simulink model "tmp_model_3"  (R2018b)
settings: Solver=VariableStepAuto  StartTime=0.0  StopTime=100  FixedStep=0.001  RelTol=1e-3
undefined symbols (not defined in the file or in its folder): GeRa
libraries: fl_lib x63, sdl_lib x20, nesl_utility x11
(part 3 of 3)

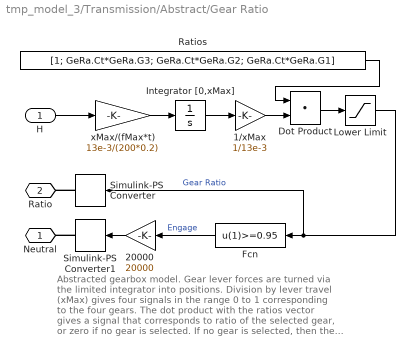
== system tmp_model_3/Transmission/Abstract/Gear Ratio ==
  note: Abstracted gearbox model. Gear lever forces are turned
      | via the limited integrator into positions. Division
      | by lever travel (xMax) gives four signals in the range
      | 0 to 1 corresponding to the four gears. The dot
      | product with the ratios vector gives a signal that
      | corresponds to ratio of the selected gear, or zero if
      | no gear is selected. If no gear is selected, then the
      | clutch is disengaged to represent neutral.
  H : Inport
  1/xMax : Gain  Gain=1/13e-3  SaturateOnIntegerOverflow=on  OutDataTypeStr=Inherit: Same as input  ParamDataTypeStr=Inherit: Same as input
  20000 : Gain  Gain=20000  SaturateOnIntegerOverflow=on  OutDataTypeStr=Inherit: Same as input  ParamDataTypeStr=Inherit: Same as input
  Dot Product : DotProduct  OutDataTypeStr=Inherit: Inherit via internal rule
  Fcn : Fcn  Expr=u(1)>=0.95
  Integrator [0,xMax] : Integrator  LimitOutput=on  UpperSaturationLimit=13e-3  LowerSaturationLimit=0
  Lower Limit : Saturate  UpperLimit=inf  LowerLimit=0.9
  Ratios : Constant  Value=[1; GeRa.Ct*GeRa.G3; GeRa.Ct*GeRa.G2; GeRa.Ct*GeRa.G1]  VectorParams1D=off
  Simulink-PS Converter : nesl_utility/Simulink-PS Converter  PhysicalDomain=network_engine_domain  SubClassName=ps_input  LeftPortType=input  RightPortType=output  PseudoPeriodic=off  Frequencies=[]  NoiseDistribution=none  NoiseParameters=[]  Unit=1  AffineConversion=off  FilteringAndDerivatives=zero  SimscapeFilterOrder=1  InputFilterTimeConstant=.001  UdotUserProvided=0
  Simulink-PS Converter1 : nesl_utility/Simulink-PS Converter  PhysicalDomain=network_engine_domain  SubClassName=ps_input  LeftPortType=input  RightPortType=output  PseudoPeriodic=off  Frequencies=[]  NoiseDistribution=none  NoiseParameters=[]  Unit=1  AffineConversion=off  FilteringAndDerivatives=zero  SimscapeFilterOrder=1  InputFilterTimeConstant=.001  UdotUserProvided=0
  xMax/(fMax*t) : Gain  Gain=13e-3/(200*0.2)  SaturateOnIntegerOverflow=on  OutDataTypeStr=Inherit: Same as input  ParamDataTypeStr=Inherit: Same as input
  Neutral : PMIOPort  Side=Right
  Ratio : PMIOPort  Port=2  Side=Right
  wires:
  Lower Limit/1 -> Fcn/1, Simulink-PS Converter/1  "Gear Ratio"
  20000/1 -> Simulink-PS Converter1/1
  Fcn/1 -> 20000/1  "Engage"
  xMax/(fMax*t)/1 -> Integrator [0,xMax]/1
  1/xMax/1 -> Dot Product/2
  Integrator [0,xMax]/1 -> 1/xMax/1
  Dot Product/1 -> Lower Limit/1
  H/1 -> xMax/(fMax*t)/1
  Ratios/1 -> Dot Product/1
  connections:
  Simulink-PS Converter1/RConn1 -- Neutral/RConn1
  Simulink-PS Converter/RConn1 -- Ratio/RConn1

== system tmp_model_3/Transmission/Detailed/Gearbox Schematic ==

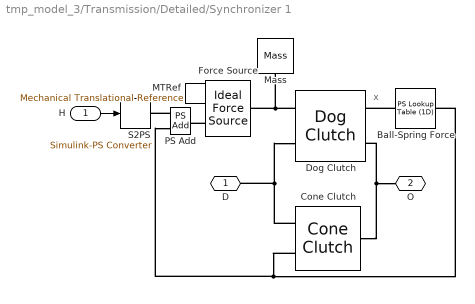
== system tmp_model_3/Transmission/Detailed/Synchronizer 1 ==
  note: x
  H : Inport
  Ball-Spring Force : fl_lib/Physical Signals/Lookup Tables/PS Lookup Table (1D)  x=[ -2 -0.1 0 0.1 2 ]*1e-3+3.2e-3  f=[ 0 100 0 -100 0 ]  interp_method=1  extrap_method=2
      settings: SourceProductName=Simscape  SourceProductBaseCode=SS
  Cone Clutch : sdl_lib/Clutches/Cone Clutch  d_o=60 mm  d_i=50 mm  theta=15 deg  friction_model=1  mu_coulomb=0.5  mu_w_vector=[ 0 0.1 0.2 0.3 0.4 0.5 1 2 5 10 100 1000 ] rad/s  mu_coulomb_vector=[ 0.29 0.28 0.26 0.22 0.21 0.2 0.2 0.19 0.19 0.19 0.19 0.19 ]  mu_interp_method=1  mu_extrap_method=1  mu_static=0.52  w_tol=0.01 rad/s  force_min=1 N  initial_state_locked=0  temperature_TLU=[280.0, 300.0, 320.0] K  mu_coulomb_temp_vector=[0.3, 0.28, 0.25]  mu_coulomb_matrix=[0.34, 0.32, 0.3; 0.3, 0.28, 0.25; 0.25, 0.2, 0.15]  mu_static_vector=[0.4, 0.38, 0.36]  thermal_mass=25 kJ/K  T_init=300 K
      settings: SourceProductName=Simscape Driveline  SourceProductBaseCode=LD
  Dog Clutch : sdl_lib/Clutches/Dog Clutch  model=2  max_torque=1000 N*m  n_teeth=6  clutch_backlash=20 deg  tooth_height=10 mm  radius=50 mm  back_stop=1  ring_hub_gap=3 mm  clutch_stiffness=1e5 N*m/rad  clutch_damping=2000 N*m/(rad/s)  transl_stiffness=1e+7 N/m  transl_damping=1000 N/(m/s)  visc_fric_transl=10 N/(m/s)  fric_coeff=1e-7  direction=1  engagement_velocity=200 rpm  engagement_overlap=1 mm  initial_state_engaged=0  init_pos=0 mm  init_rel_angle=0 deg  temperature_TLU=[280.0, 300.0, 320.0] K  max_torque_vector=[1000.0, 1050.0, 1000.0] N*m  interp_method=1  extrap_method=1  thermal_mass=25 kJ/K  T_init=300 K
      settings: SourceProductName=Simscape Driveline  SourceProductBaseCode=LD
  Force Source : fl_lib/Mechanical/Mechanical Sources/Ideal Force Source
  MTRef : fl_lib/Mechanical/Translational Elements/Mechanical Translational Reference
  Mass : fl_lib/Mechanical/Translational Elements/Mass  mass=0.1 kg  v_specify=off  v_priority=High  v=0 m/s  v_nominal_specify=off  v_nominal_unit=m/s  v_nominal_value=1  f_specify=off  f_priority=High  f=0 N  f_nominal_specify=off  f_nominal_unit=N  f_nominal_value=1
  PS Add : fl_lib/Physical Signals/Functions/PS Add
  S2PS : nesl_utility/Simulink-PS Converter  PhysicalDomain=network_engine_domain  SubClassName=ps_input  LeftPortType=input  RightPortType=output  PseudoPeriodic=off  Frequencies=[]  NoiseDistribution=none  NoiseParameters=[]  Unit=1  AffineConversion=off  FilteringAndDerivatives=zero  SimscapeFilterOrder=1  InputFilterTimeConstant=.001  UdotUserProvided=1
  D : PMIOPort  Side=Left
  O : PMIOPort  Port=2  Side=Right
  wires:
  H/1 -> S2PS/1
  connections:
  PS Add/LConn1 -- S2PS/RConn1
  Dog Clutch/LConn1 -- Force Source/LConn1 -- Mass/LConn1
  D/RConn1 -- Cone Clutch/LConn2 -- Dog Clutch/LConn2
  Cone Clutch/RConn1 -- Dog Clutch/RConn2 -- O/RConn1
  Cone Clutch/LConn1 -- Ball-Spring Force/RConn1 -- PS Add/LConn2
  Ball-Spring Force/LConn1 -- Dog Clutch/RConn1
  MTRef/LConn1 -- Force Source/RConn2
  Force Source/RConn1 -- PS Add/RConn1

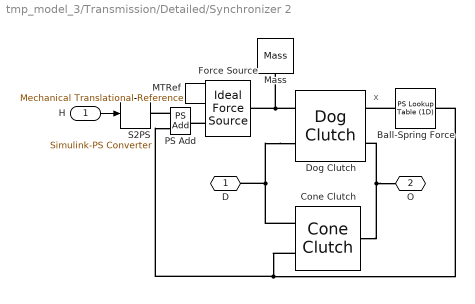
== system tmp_model_3/Transmission/Detailed/Synchronizer 2 ==
  note: x
  H : Inport
  Ball-Spring Force : fl_lib/Physical Signals/Lookup Tables/PS Lookup Table (1D)  x=[ -2 -0.1 0 0.1 2 ]*1e-3+3.2e-3  f=[ 0 100 0 -100 0 ]  interp_method=1  extrap_method=2
      settings: SourceProductName=Simscape  SourceProductBaseCode=SS
  Cone Clutch : sdl_lib/Clutches/Cone Clutch  d_o=60 mm  d_i=50 mm  theta=15 deg  friction_model=1  mu_coulomb=0.5  mu_w_vector=[ 0 0.1 0.2 0.3 0.4 0.5 1 2 5 10 100 1000 ] rad/s  mu_coulomb_vector=[ 0.29 0.28 0.26 0.22 0.21 0.2 0.2 0.19 0.19 0.19 0.19 0.19 ]  mu_interp_method=1  mu_extrap_method=1  mu_static=0.52  w_tol=0.01 rad/s  force_min=1 N  initial_state_locked=0  temperature_TLU=[280.0, 300.0, 320.0] K  mu_coulomb_temp_vector=[0.3, 0.28, 0.25]  mu_coulomb_matrix=[0.34, 0.32, 0.3; 0.3, 0.28, 0.25; 0.25, 0.2, 0.15]  mu_static_vector=[0.4, 0.38, 0.36]  thermal_mass=25 kJ/K  T_init=300 K
      settings: SourceProductName=Simscape Driveline  SourceProductBaseCode=LD
  Dog Clutch : sdl_lib/Clutches/Dog Clutch  model=2  max_torque=1000 N*m  n_teeth=6  clutch_backlash=20 deg  tooth_height=10 mm  radius=50 mm  back_stop=1  ring_hub_gap=3 mm  clutch_stiffness=1e5 N*m/rad  clutch_damping=2000 N*m/(rad/s)  transl_stiffness=1e+7 N/m  transl_damping=1000 N/(m/s)  visc_fric_transl=10 N/(m/s)  fric_coeff=1e-7  direction=1  engagement_velocity=200 rpm  engagement_overlap=1 mm  initial_state_engaged=0  init_pos=0 mm  init_rel_angle=0 deg  temperature_TLU=[280.0, 300.0, 320.0] K  max_torque_vector=[1000.0, 1050.0, 1000.0] N*m  interp_method=1  extrap_method=1  thermal_mass=25 kJ/K  T_init=300 K
      settings: SourceProductName=Simscape Driveline  SourceProductBaseCode=LD
  Force Source : fl_lib/Mechanical/Mechanical Sources/Ideal Force Source
  MTRef : fl_lib/Mechanical/Translational Elements/Mechanical Translational Reference
  Mass : fl_lib/Mechanical/Translational Elements/Mass  mass=0.1 kg  v_specify=off  v_priority=High  v=0 m/s  v_nominal_specify=off  v_nominal_unit=m/s  v_nominal_value=1  f_specify=off  f_priority=High  f=0 N  f_nominal_specify=off  f_nominal_unit=N  f_nominal_value=1
  PS Add : fl_lib/Physical Signals/Functions/PS Add
  S2PS : nesl_utility/Simulink-PS Converter  PhysicalDomain=network_engine_domain  SubClassName=ps_input  LeftPortType=input  RightPortType=output  PseudoPeriodic=off  Frequencies=[]  NoiseDistribution=none  NoiseParameters=[]  Unit=1  AffineConversion=off  FilteringAndDerivatives=zero  SimscapeFilterOrder=1  InputFilterTimeConstant=.001  UdotUserProvided=1
  D : PMIOPort  Side=Left
  O : PMIOPort  Port=2  Side=Right
  wires:
  H/1 -> S2PS/1
  connections:
  Force Source/RConn1 -- PS Add/RConn1
  MTRef/LConn1 -- Force Source/RConn2
  Ball-Spring Force/LConn1 -- Dog Clutch/RConn1
  Ball-Spring Force/RConn1 -- PS Add/LConn2 -- Cone Clutch/LConn1
  O/RConn1 -- Dog Clutch/RConn2 -- Cone Clutch/RConn1
  Dog Clutch/LConn2 -- D/RConn1 -- Cone Clutch/LConn2
  Force Source/LConn1 -- Mass/LConn1 -- Dog Clutch/LConn1
  PS Add/LConn1 -- S2PS/RConn1

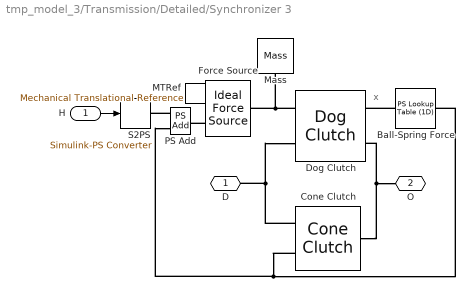
== system tmp_model_3/Transmission/Detailed/Synchronizer 3 ==
  note: x
  H : Inport
  Ball-Spring Force : fl_lib/Physical Signals/Lookup Tables/PS Lookup Table (1D)  x=[ -2 -0.1 0 0.1 2 ]*1e-3+3.2e-3  f=[ 0 100 0 -100 0 ]  interp_method=1  extrap_method=2
      settings: SourceProductName=Simscape  SourceProductBaseCode=SS
  Cone Clutch : sdl_lib/Clutches/Cone Clutch  d_o=60 mm  d_i=50 mm  theta=15 deg  friction_model=1  mu_coulomb=0.5  mu_w_vector=[ 0 0.1 0.2 0.3 0.4 0.5 1 2 5 10 100 1000 ] rad/s  mu_coulomb_vector=[ 0.29 0.28 0.26 0.22 0.21 0.2 0.2 0.19 0.19 0.19 0.19 0.19 ]  mu_interp_method=1  mu_extrap_method=1  mu_static=0.52  w_tol=0.01 rad/s  force_min=1 N  initial_state_locked=0  temperature_TLU=[280.0, 300.0, 320.0] K  mu_coulomb_temp_vector=[0.3, 0.28, 0.25]  mu_coulomb_matrix=[0.34, 0.32, 0.3; 0.3, 0.28, 0.25; 0.25, 0.2, 0.15]  mu_static_vector=[0.4, 0.38, 0.36]  thermal_mass=25 kJ/K  T_init=300 K
      settings: SourceProductName=Simscape Driveline  SourceProductBaseCode=LD
  Dog Clutch : sdl_lib/Clutches/Dog Clutch  model=2  max_torque=1000 N*m  n_teeth=6  clutch_backlash=20 deg  tooth_height=10 mm  radius=50 mm  back_stop=1  ring_hub_gap=3 mm  clutch_stiffness=1e5 N*m/rad  clutch_damping=2000 N*m/(rad/s)  transl_stiffness=1e+7 N/m  transl_damping=1000 N/(m/s)  visc_fric_transl=10 N/(m/s)  fric_coeff=1e-7  direction=1  engagement_velocity=200 rpm  engagement_overlap=1 mm  initial_state_engaged=0  init_pos=0 mm  init_rel_angle=0 deg  temperature_TLU=[280.0, 300.0, 320.0] K  max_torque_vector=[1000.0, 1050.0, 1000.0] N*m  interp_method=1  extrap_method=1  thermal_mass=25 kJ/K  T_init=300 K
      settings: SourceProductName=Simscape Driveline  SourceProductBaseCode=LD
  Force Source : fl_lib/Mechanical/Mechanical Sources/Ideal Force Source
  MTRef : fl_lib/Mechanical/Translational Elements/Mechanical Translational Reference
  Mass : fl_lib/Mechanical/Translational Elements/Mass  mass=0.1 kg  v_specify=off  v_priority=High  v=0 m/s  v_nominal_specify=off  v_nominal_unit=m/s  v_nominal_value=1  f_specify=off  f_priority=High  f=0 N  f_nominal_specify=off  f_nominal_unit=N  f_nominal_value=1
  PS Add : fl_lib/Physical Signals/Functions/PS Add
  S2PS : nesl_utility/Simulink-PS Converter  PhysicalDomain=network_engine_domain  SubClassName=ps_input  LeftPortType=input  RightPortType=output  PseudoPeriodic=off  Frequencies=[]  NoiseDistribution=none  NoiseParameters=[]  Unit=1  AffineConversion=off  FilteringAndDerivatives=zero  SimscapeFilterOrder=1  InputFilterTimeConstant=.001  UdotUserProvided=1
  D : PMIOPort  Side=Left
  O : PMIOPort  Port=2  Side=Right
  wires:
  H/1 -> S2PS/1
  connections:
  PS Add/LConn1 -- S2PS/RConn1
  Dog Clutch/LConn1 -- Mass/LConn1 -- Force Source/LConn1
  Cone Clutch/LConn2 -- D/RConn1 -- Dog Clutch/LConn2
  Cone Clutch/RConn1 -- Dog Clutch/RConn2 -- O/RConn1
  Cone Clutch/LConn1 -- PS Add/LConn2 -- Ball-Spring Force/RConn1
  Ball-Spring Force/LConn1 -- Dog Clutch/RConn1
  MTRef/LConn1 -- Force Source/RConn2
  Force Source/RConn1 -- PS Add/RConn1

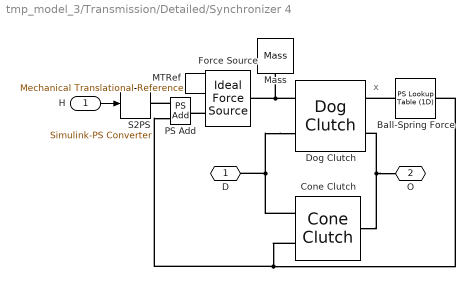
== system tmp_model_3/Transmission/Detailed/Synchronizer 4 ==
  note: x
  H : Inport
  Ball-Spring Force : fl_lib/Physical Signals/Lookup Tables/PS Lookup Table (1D)  x=[ -2 -0.1 0 0.1 2 ]*1e-3+3.2e-3  f=[ 0 100 0 -100 0 ]  interp_method=1  extrap_method=2
      settings: SourceProductName=Simscape  SourceProductBaseCode=SS
  Cone Clutch : sdl_lib/Clutches/Cone Clutch  d_o=60 mm  d_i=50 mm  theta=15 deg  friction_model=1  mu_coulomb=0.5  mu_w_vector=[ 0 0.1 0.2 0.3 0.4 0.5 1 2 5 10 100 1000 ] rad/s  mu_coulomb_vector=[ 0.29 0.28 0.26 0.22 0.21 0.2 0.2 0.19 0.19 0.19 0.19 0.19 ]  mu_interp_method=1  mu_extrap_method=1  mu_static=0.52  w_tol=0.01 rad/s  force_min=1 N  initial_state_locked=0  temperature_TLU=[280.0, 300.0, 320.0] K  mu_coulomb_temp_vector=[0.3, 0.28, 0.25]  mu_coulomb_matrix=[0.34, 0.32, 0.3; 0.3, 0.28, 0.25; 0.25, 0.2, 0.15]  mu_static_vector=[0.4, 0.38, 0.36]  thermal_mass=25 kJ/K  T_init=300 K
      settings: SourceProductName=Simscape Driveline  SourceProductBaseCode=LD
  Dog Clutch : sdl_lib/Clutches/Dog Clutch  model=2  max_torque=1000 N*m  n_teeth=6  clutch_backlash=20 deg  tooth_height=10 mm  radius=50 mm  back_stop=1  ring_hub_gap=3 mm  clutch_stiffness=1e5 N*m/rad  clutch_damping=2000 N*m/(rad/s)  transl_stiffness=1e+7 N/m  transl_damping=1000 N/(m/s)  visc_fric_transl=10 N/(m/s)  fric_coeff=1e-7  direction=1  engagement_velocity=200 rpm  engagement_overlap=1 mm  initial_state_engaged=0  init_pos=0 mm  init_rel_angle=0 deg  temperature_TLU=[280.0, 300.0, 320.0] K  max_torque_vector=[1000.0, 1050.0, 1000.0] N*m  interp_method=1  extrap_method=1  thermal_mass=25 kJ/K  T_init=300 K
      settings: SourceProductName=Simscape Driveline  SourceProductBaseCode=LD
  Force Source : fl_lib/Mechanical/Mechanical Sources/Ideal Force Source
  MTRef : fl_lib/Mechanical/Translational Elements/Mechanical Translational Reference
  Mass : fl_lib/Mechanical/Translational Elements/Mass  mass=0.1 kg  v_specify=off  v_priority=High  v=0 m/s  v_nominal_specify=off  v_nominal_unit=m/s  v_nominal_value=1  f_specify=off  f_priority=High  f=0 N  f_nominal_specify=off  f_nominal_unit=N  f_nominal_value=1
  PS Add : fl_lib/Physical Signals/Functions/PS Add
  S2PS : nesl_utility/Simulink-PS Converter  PhysicalDomain=network_engine_domain  SubClassName=ps_input  LeftPortType=input  RightPortType=output  PseudoPeriodic=off  Frequencies=[]  NoiseDistribution=none  NoiseParameters=[]  Unit=1  AffineConversion=off  FilteringAndDerivatives=zero  SimscapeFilterOrder=1  InputFilterTimeConstant=.001  UdotUserProvided=1
  D : PMIOPort  Side=Left
  O : PMIOPort  Port=2  Side=Right
  wires:
  H/1 -> S2PS/1
  connections:
  Force Source/RConn1 -- PS Add/RConn1
  MTRef/LConn1 -- Force Source/RConn2
  Ball-Spring Force/LConn1 -- Dog Clutch/RConn1
  Ball-Spring Force/RConn1 -- PS Add/LConn2 -- Cone Clutch/LConn1
  O/RConn1 -- Dog Clutch/RConn2 -- Cone Clutch/RConn1
  Dog Clutch/LConn2 -- D/RConn1 -- Cone Clutch/LConn2
  Force Source/LConn1 -- Mass/LConn1 -- Dog Clutch/LConn1
  PS Add/LConn1 -- S2PS/RConn1

== matlab function tmp_model_3/State1 ==
  data: y4 output; y3 output; y2 output; u1 input; y1 output; u2 input; clutch output; gas output; it input; TClutch input; TGas input; TSynchron input
function [y4,y3,y2,y1, clutch, gas] = fcn(u1, u2, it, TClutch, TGas, TSynchron)

clutch = 0.0;
gas = 0.0;
y1 = 0;
y2 = 0;
y3 = 0;
y4 = 0;

if (it < 0.3)
    clutch = 0;
    gas = 0.0;
    y1 = 0;
    y2 = 0;
    y3 = 0;
    y4 = 0;
else 
    if (it > 1) && (it < 2.5)  % I
        clutch = 120;
        y1 = 200;
        y2 = 0;
        y3 = 0;
        y4 = 0;
        return;
    end

    if (it > 2.5) && (it < 2.6)  % I
        clutch = 90;
        return;
    end
    
    if (it > 2.6) && (it < 2.7)  % I
        clutch = 60;
        return;
    end
    
    if (it > 2.7) && (it < 2.8)  % I
        clutch = 30;
        return;
    end    
    
    if(it > 2.7) && (it < 3.5)
    %if(u1 > 2600 && u1 < 3000)   GAS
        gas = 1; %0.7
    end

    if (it > 6) && (it < 7)
%     if(u1 > 4000 && u1 < 5000)  % -I
        gas = 0;
        y1 = -200;
        y3 = 0;
        y4 = 0;
    end

    if(it > 6.7) && (it < 7.5)  % II
%     if(u1 > 3000 && u1 < 4000)  % II
        clutch = 120;
        gas = 0.0;
        y2 = 200;
        y3 = 0;
        y4 = 0;
        return;
    end
    
    if(it > 7.5) && (it < 7.6)
        clutch = 90;
        return;
    end    
    
    if(it > 7.6) && (it < 7.7)
        clutch = 60;
        return;
    end    
    
    if(it > 7.7) && (it < 7.8)
        clutch = 30;
        return;
    end
    
    if(it > 7.6) && (it < 11.5)  % GAS 10.2
        gas = 1.0;
    end

    if(it > 11.5 + 3) && (it < 12.5 + 3)  % -II
        gas = 0;
        y2 = -200;
        y1 = 0;
        y4 = 0;
    end   

%     if(u1 > 4000 && u1 < 5000)  % III
    if(it > 12 +3) && (it < 13 + 3)
        clutch = 120;
        gas = 0.0;
        y3 = 200;
        y1 = 0;
        y4 = 0;
        return;
    end

    if(it > 13 +3) && (it < 13.1 +3)
        clutch = 90;
        return;
    end
    
    if(it > 13.1+3) && (it < 13.2+3)
        clutch = 60;
        return;
    end
    
    if(it > 13.2+3) && (it < 13.3+3)
        clutch = 30;
        return;
    end
    
    
    if(it > 13.3+3) && (it < 14.3 + 3 + 1.5 + 5 + 3.5 )  % GAS 13.6
        gas = 1.0;
    end
    
    if(it > 16+5+3+10) && (it < 17+5+3+10)  % -III
        gas = 0;
        y3 = -200;
        y1 = 0;
        y4 = 0;
    end 
    
    if(it > 16.5+5+3+10) && (it < 17.5+5+3+10)    % IV
        clutch = 120;
        gas = 0.0;
        y4 = 200;
        y1 = 0;
        y2 = 0;
        return;
    end
    
    if(it > 17.5+5+3+10) && (it < 17.6+5+3+10)    % IV
        clutch = 90;
        return;
    end

    if(it > 17.6+5+3+10) && (it < 17.7+5+3+10)    % IV
        clutch = 60;
        return;
    end
    
    if(it > 17.7+5+3+10) && (it < 17.8+5+3+10)    % IV
        clutch = 30;
        return;
    end
    
    if(it > 17.8+5+3+10) && (it < 18+5+3+10+7)  % GAS
        gas = 1.0;
    end
    if(it > 18+5+3+10+7) && (it < 18+5+3+10+7+20)  % GAS
        gas = 0.2;
    end
    
%     if(it > 21) && (it < 22)  % -IV
%         gas = 0;
%         y4 = -200;
%         y1 = 0;
%         y2 = 0;
%     end 
    
end
